simulink library "PC_GS_SSMB"  (R2024a)
settings: Solver=VariableStepAuto  StartTime=0.0  StopTime=10.0  RelTol=1e-3
undefined symbols (not defined in the file): points, X, Y, Z, z_query
libraries: sm_lib x22
settings Model: Creator=jjansev  LastModifiedBy=jjansev

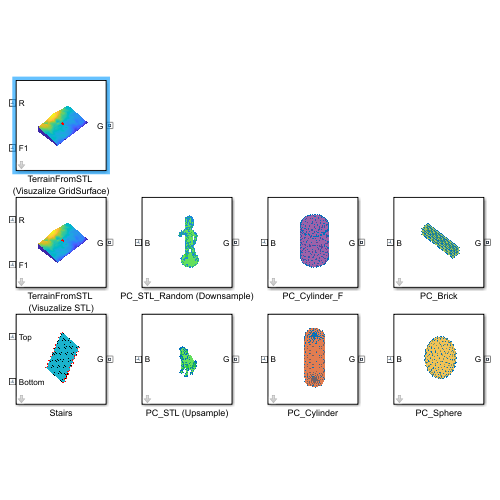
[thumbnail: Simulink's stored preview of the top-level diagram]
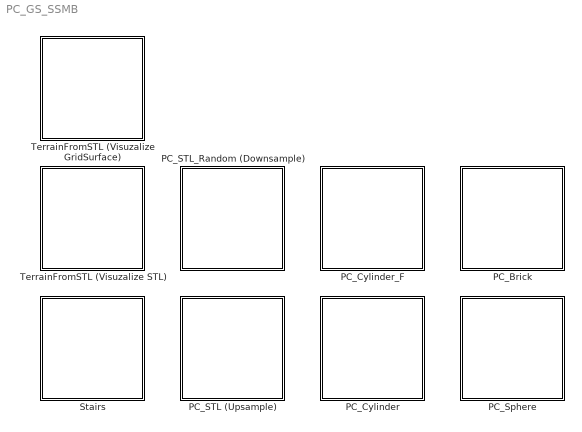
== system PC_GS_SSMB ==
  PC_Brick : Subsystem  mask{length=250, width=50, height=30, numDivisionsLength=25, numDivisionsWidth=5, numDivisionsHeight=3, patchColor=[0.4660, 0.6740, 0.1880], markerColor=[0 0.4470 0.7410]}
      mask prompts: length "Length of the brick (x) [mm]"; width "Width of the brick (y) [mm]"; height "Height of the brick (z) [mm]"; numDivisionsLength "Number of divisions along the length"; numDivisionsWidth "Number of divisions along the width"; numDivisionsHeight "Number of divisions along the height"; patchColor "Color of the patches"; markerColor "Color of the markers"
      mask init:
      | [points, imageMatrix] = generateBrickPointCloud(length, width, height, numDivisionsLength, numDivisionsWidth, numDivisionsHeight, patchColor, markerColor);
      mask Display: image(imageMatrix);
  PC_Cylinder : Subsystem  mask{radius=51, height=200, numRadialDivisions=5, angularOffset=pi/5, numHeightDivisions=25, numFaceRadialDivisions=10, faceAngularOffset=pi/10, numFaceAngularDivisions=10, patchColor=[0.8500, 0.3250, 0.0980], markerColor=[0 0.4470 0.7410]}
      mask prompts: radius "Radius of the cylider [mm]"; height "Height of the cylinder [mm]"; numRadialDivisions "Number of divisions around the circumference"; angularOffset "Angular offset in radians for each layer"; numHeightDivisions "Number of divisions along the height"; numFaceRadialDivisions "Number of radial divisions for the circular faces"; numFaceAngularDivisions "Number of angular divisions for the circular faces"; patchColor "RGB color for the patches"; markerColor "RGB color for the markers"
      mask init:
      | [points, imageMatrix] = generateCylinderPointCloud(radius, height, numRadialDivisions, numHeightDivisions, numFaceRadialDivisions, numFaceAngularDivisions, angularOffset, faceAngularOffset, patchColor, markerColor);
      mask Display: image(imageMatrix);
  PC_Cylinder_F : Subsystem  mask{radius=150/2, height=150, numPoints=150, numCircumferencePoints=50, numFacePoints=50, patchColor=[0.4940, 0.1840, 0.5560], markerColor=[0 0.4470 0.7410]}
      mask prompts: radius "Radius of the cylider [mm]"; height "Height of the cylinder [mm]"; numPoints "Total number of points for the curved surface using the Fibonacci lattice"; numCircumferencePoints "Number of points on the circumference of each disc"; numFacePoints "Number of points on each disc surface using the Fibonacci lattice"; patchColor "RGB color for the patches"; markerColor "RGB color for the markers"
      mask init:
      | [points, imageMatrix] = generateCylinderPointCloudFibonacci(radius, height, numPoints, numCircumferencePoints, numFacePoints, patchColor, markerColor);
      mask Display: image(imageMatrix);
  PC_STL (Upsample) : Subsystem  mask{stlFilename='Low_Poly_Pug.STL', numPoints=0, patchColor=[0.1940, 0.840, 0.1560], markerColor=[0 0.4470 0.7410], STL_points=on}
      mask prompts: stlFilename "Path to the STL file"; numPoints "Number of Points to add inbetween the vertices of the STL"; patchColor "RGB color for the patches"; markerColor "RGB color for the markers"; STL_points "Should the Original STL Points be included in the Point Cloud"
      mask init:
      | % Use set_param to set the parameter
      | fileSolidName = [gcb, '/File Solid'];
      | set_param(fileSolidName, 'ExtGeomFileName', stlFilename);
      | 
      | [points, imageMatrix] = generateSTLPointCloud(stlFilename, numPoints, patchColor, markerColor, STL_points);
      mask Display: image(imageMatrix);
  PC_STL_Random (Downsample) : Subsystem  mask{stlFilename='VaultBoy.STL', numPoints=0, patchColor=[0.1940, 0.840, 0.1560], markerColor=[0.1 0.5470 0.8410], STL_points=on, numPoints2=500}
      mask prompts: stlFilename "Path to the STL file"; numPoints "Points to be added into large surfaces"; patchColor "RGB color for the patches"; markerColor "RGB color for the markers"; STL_points "Should a Subset of the Original STL Points be included in the Point Cloud"; numPoints2 "How many points should be randomly added"
      mask init:
      | % Use set_param to set the parameter
      | fileSolidName = [gcb, '/File Solid'];
      | set_param(fileSolidName, 'ExtGeomFileName', stlFilename);
      | 
      | [points, imageMatrix] = generateSTLPointCloudRandom(stlFilename, numPoints, patchColor, markerColor, STL_points, numPoints2);
      mask Display: image(imageMatrix);
  PC_Sphere : Subsystem  mask{numPoints=256, radius=50, patchColor=[0.9290, 0.6940, 0.1250], markerColor=[0 0.4470 0.7410], dens=1}
      mask prompts: numPoints "Number of points on the Surface of the Sphere"; radius "Radius of the Sphere [mm]"; patchColor "Color of the patches"; markerColor "Color of the markers"; dens "Density"
      mask init:
      | [points, imageMatrix] = generateSpherePointCloud(numPoints, radius, patchColor, markerColor);
      mask Display: image(imageMatrix);
  Stairs : Subsystem  mask{nSteps=10, Tread=180, NosingProtusion=35, Riser=180, yWidth=2000, input_angle_degrees=-45, markerColor=[1 0 0], patchColor=[0.1 0.7 0.8]}
      mask prompts: nSteps "Number of steps"; Tread "Tread [mm]"; NosingProtusion "Nosing Protusion [mm]"; Riser "Riser [mm]"; yWidth "Width of the Staircase"; input_angle_degrees "Degrees to rotate to ensure a single z value per x value [deg]"; markerColor "Color of the markers in the mask image"; patchColor "Surface color"
      mask init:
      | [X_grid_vector, Y_grid_vector, Z_heights, imageMatrix, x, z] = generateStaircaseSurface(nSteps, Tread, NosingProtusion, Riser, yWidth, input_angle_degrees, markerColor, patchColor);
      mask Display: image(imageMatrix);
  TerrainFromSTL (Visuzalize GridSurface) : Subsystem  mask{stlFileName='MRC_t.stl', resolution=1, color=[0.5 0.5 0.6], x_query=0, y_query=0, Int_method=Linear}
      mask prompts: stlFileName "STL Filename"; resolution "Resolution of the Grid surface [m]"; color "Color of the Grid-surface"; x_query "Position on x-axis to be polled for z-height (Frame F1)"; y_query "Position on y-axis to be polled for z-height (Frame F1)"; Int_method "Interpolation method Used of the Surface"
      mask init:
      | % Use set_param to set the parameter
      | fileSolidName = [gcb, '/File Solid'];
      | set_param(fileSolidName, 'ExtGeomFileName', stlFileName);
      | 
      | [imageMatrix, xi, yi, ZI, Res_orig, z_query] = GenerateTerrainFromSTL(stlFileName, resolution, x_query, y_query, Int_method);
      mask Display: image(imageMatrix);
  TerrainFromSTL (Visuzalize STL) : Subsystem  mask{stlFileName='MRC_t.stl', resolution=1, color=[0.5 0.5 0.6], x_query=0, y_query=0, Int_method=Linear}
      mask prompts: stlFileName "STL Filename"; resolution "Resolution of the Grid surface [m]"; color "Color of the Grid-surface"; x_query "Position on x-axis to be polled for z-height (Frame F1)"; y_query "Position on y-axis to be polled for z-height (Frame F1)"; Int_method "Interpolation method Used of the Surface"
      mask init: same as PC_GS_SSMB/TerrainFromSTL (Visuzalize GridSurface)
      mask Display: image(imageMatrix);

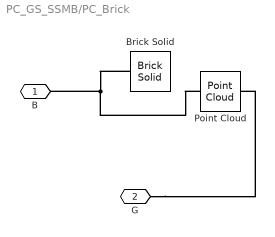
== system PC_GS_SSMB/PC_Brick ==
  Brick Solid : sm_lib/Body Elements/Brick Solid  BrickDimensions=[length width height]  BrickDimensionsUnits=mm  ExportEntireGeometry=off  InertiaType=CalculateFromGeometry  BasedOnType=Density  Density=1000  DensityUnits=kg/m^3  Mass=1  MassUnits=kg  CenterOfMass=[0 0 0]  CenterOfMassUnits=m  MomentsOfInertia=[1 1 1]  MomentsOfInertiaUnits=kg*m^2  ProductsOfInertia=[0 0 0]  ProductsOfInertiaUnits=kg*m^2  GraphicType=FromGeometry  MarkerShape=Sphere  MarkerSize=10  GraphicVisPropType=SimpleVisualProperties  GraphicDiffuseColor=patchColor  GraphicOpacity=0.85  GraphicSpecularColor=[0.5 0.5 0.5 1.0]  GraphicAmbientColor=[0.15 0.15 0.15 1.0]  GraphicEmissiveColor=[0.0 0.0 0.0 1.0]  GraphicShininess=75  DoExposeReferenceFrame=on  SerializedFrames=<Frames/>
  Point Cloud : sm_lib/Curves and Surfaces/Point Cloud  CoordinatesMatrix=points  CoordinatesMatrixUnits=mm  GraphicType=MarkerCloud  GraphicSphereRadius=max(max(points)-min(points))/100*2  GraphicSphereRadiusUnits=mm  GraphicVisPropType=SimpleVisualProperties  GraphicDiffuseColor=markerColor  GraphicOpacity=1  GraphicSpecularColor=[0.5 0.5 0.5 1.0]  GraphicAmbientColor=[0.15 0.15 0.15 1.0]  GraphicEmissiveColor=[0.0 0.0 0.0 1.0]  GraphicShininess=75
  B : PMIOPort  Side=Left
  G : PMIOPort  Port=2  Side=Right
  connections:
  G/RConn1 -- Point Cloud/RConn1
  Point Cloud/LConn1 -- B/RConn1 -- Brick Solid/RConn1

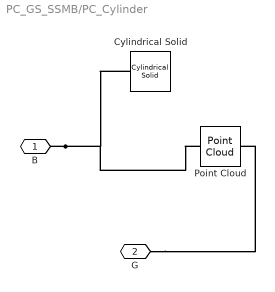
== system PC_GS_SSMB/PC_Cylinder ==
  Cylindrical Solid : sm_lib/Body Elements/Cylindrical Solid  CylinderRadius=radius  CylinderRadiusUnits=mm  CylinderLength=height  CylinderLengthUnits=mm  ExportEntireGeometry=off  InertiaType=CalculateFromGeometry  BasedOnType=Density  Density=1000  DensityUnits=kg/m^3  Mass=1  MassUnits=kg  CenterOfMass=[0 0 0]  CenterOfMassUnits=m  MomentsOfInertia=[1 1 1]  MomentsOfInertiaUnits=kg*m^2  ProductsOfInertia=[0 0 0]  ProductsOfInertiaUnits=kg*m^2  GraphicType=FromGeometry  MarkerShape=Sphere  MarkerSize=10  GraphicVisPropType=SimpleVisualProperties  GraphicDiffuseColor=patchColor  GraphicOpacity=0.85  GraphicSpecularColor=[0.5 0.5 0.5 1.0]  GraphicAmbientColor=[0.15 0.15 0.15 1.0]  GraphicEmissiveColor=[0.0 0.0 0.0 1.0]  GraphicShininess=75  DoExposeReferenceFrame=on  SerializedFrames=<Frames/>
  Point Cloud : sm_lib/Curves and Surfaces/Point Cloud  CoordinatesMatrix=points  CoordinatesMatrixUnits=mm  GraphicType=MarkerCloud  GraphicSphereRadius=max(max(points)-min(points))/100*2  GraphicSphereRadiusUnits=mm  GraphicVisPropType=SimpleVisualProperties  GraphicDiffuseColor=markerColor  GraphicOpacity=1  GraphicSpecularColor=[0.5 0.5 0.5 1.0]  GraphicAmbientColor=[0.15 0.15 0.15 1.0]  GraphicEmissiveColor=[0.0 0.0 0.0 1.0]  GraphicShininess=75
  B : PMIOPort  Side=Left
  G : PMIOPort  Port=2  Side=Right
  connections:
  B/RConn1 -- Point Cloud/LConn1 -- Cylindrical Solid/RConn1
  G/RConn1 -- Point Cloud/RConn1

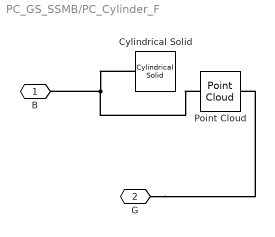
== system PC_GS_SSMB/PC_Cylinder_F ==
  Cylindrical Solid : sm_lib/Body Elements/Cylindrical Solid  CylinderRadius=radius  CylinderRadiusUnits=mm  CylinderLength=height  CylinderLengthUnits=mm  ExportEntireGeometry=off  InertiaType=CalculateFromGeometry  BasedOnType=Density  Density=1000  DensityUnits=kg/m^3  Mass=1  MassUnits=kg  CenterOfMass=[0 0 0]  CenterOfMassUnits=m  MomentsOfInertia=[1 1 1]  MomentsOfInertiaUnits=kg*m^2  ProductsOfInertia=[0 0 0]  ProductsOfInertiaUnits=kg*m^2  GraphicType=FromGeometry  MarkerShape=Sphere  MarkerSize=10  GraphicVisPropType=SimpleVisualProperties  GraphicDiffuseColor=patchColor  GraphicOpacity=0.85  GraphicSpecularColor=[0.5 0.5 0.5 1.0]  GraphicAmbientColor=[0.15 0.15 0.15 1.0]  GraphicEmissiveColor=[0.0 0.0 0.0 1.0]  GraphicShininess=75  DoExposeReferenceFrame=on  SerializedFrames=<Frames/>
  Point Cloud : sm_lib/Curves and Surfaces/Point Cloud  CoordinatesMatrix=points  CoordinatesMatrixUnits=mm  GraphicType=MarkerCloud  GraphicSphereRadius=max(max(points)-min(points))/100*2  GraphicSphereRadiusUnits=mm  GraphicVisPropType=SimpleVisualProperties  GraphicDiffuseColor=markerColor  GraphicOpacity=1  GraphicSpecularColor=[0.5 0.5 0.5 1.0]  GraphicAmbientColor=[0.15 0.15 0.15 1.0]  GraphicEmissiveColor=[0.0 0.0 0.0 1.0]  GraphicShininess=75
  B : PMIOPort  Side=Left
  G : PMIOPort  Port=2  Side=Right
  connections:
  G/RConn1 -- Point Cloud/RConn1
  Point Cloud/LConn1 -- B/RConn1 -- Cylindrical Solid/RConn1

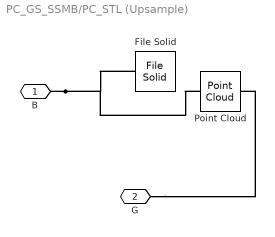
== system PC_GS_SSMB/PC_STL (Upsample) ==
  File Solid : sm_lib/Body Elements/File Solid  ExtGeomFileName=Low_Poly_Pug.STL  UnitType=Custom  ExtGeomFileUnits=mm  StepReaderType=HEX  ExportConvexHullGeometry=off  InertiaType=CalculateFromGeometry  BasedOnType=Density  Density=7850  DensityUnits=kg/m^3  Mass=1  MassUnits=kg  CenterOfMass=[0 0 0]  CenterOfMassUnits=m  MomentsOfInertia=[1 1 1]  MomentsOfInertiaUnits=kg*m^2  ProductsOfInertia=[0 0 0]  ProductsOfInertiaUnits=kg*m^2  GraphicType=FromGeometry  MarkerShape=Sphere  MarkerSize=10  GraphicVisPropType=SimpleVisualProperties  GraphicDiffuseColor=patchColor  GraphicOpacity=1  GraphicSpecularColor=[0.5 0.5 0.5 1.0]  GraphicAmbientColor=[0.15 0.15 0.15 1.0]  GraphicEmissiveColor=[0.0 0.0 0.0 1.0]  GraphicShininess=75  DoExposeReferenceFrame=on  SerializedFrames=<Frames/>
  Point Cloud : sm_lib/Curves and Surfaces/Point Cloud  CoordinatesMatrix=points  CoordinatesMatrixUnits=mm  GraphicType=MarkerCloud  GraphicSphereRadius=max(max(points)-min(points))/100*2  GraphicSphereRadiusUnits=mm  GraphicVisPropType=SimpleVisualProperties  GraphicDiffuseColor=markerColor  GraphicOpacity=1  GraphicSpecularColor=[0.5 0.5 0.5 1.0]  GraphicAmbientColor=[0.15 0.15 0.15 1.0]  GraphicEmissiveColor=[0.0 0.0 0.0 1.0]  GraphicShininess=75
  B : PMIOPort  Side=Left
  G : PMIOPort  Port=2  Side=Right
  connections:
  B/RConn1 -- Point Cloud/LConn1 -- File Solid/RConn1
  G/RConn1 -- Point Cloud/RConn1

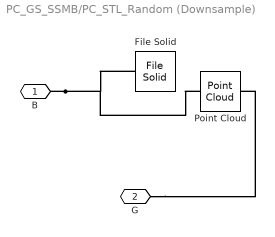
== system PC_GS_SSMB/PC_STL_Random (Downsample) ==
  File Solid : sm_lib/Body Elements/File Solid  ExtGeomFileName=VaultBoy.STL  UnitType=Custom  ExtGeomFileUnits=mm  StepReaderType=HEX  ExportConvexHullGeometry=off  InertiaType=CalculateFromGeometry  BasedOnType=Density  Density=7850  DensityUnits=kg/m^3  Mass=1  MassUnits=kg  CenterOfMass=[0 0 0]  CenterOfMassUnits=m  MomentsOfInertia=[1 1 1]  MomentsOfInertiaUnits=kg*m^2  ProductsOfInertia=[0 0 0]  ProductsOfInertiaUnits=kg*m^2  GraphicType=FromGeometry  MarkerShape=Sphere  MarkerSize=10  GraphicVisPropType=SimpleVisualProperties  GraphicDiffuseColor=patchColor  GraphicOpacity=1  GraphicSpecularColor=[0.5 0.5 0.5 1.0]  GraphicAmbientColor=[0.15 0.15 0.15 1.0]  GraphicEmissiveColor=[0.0 0.0 0.0 1.0]  GraphicShininess=75  DoExposeReferenceFrame=on  SerializedFrames=<Frames/>
  Point Cloud : sm_lib/Curves and Surfaces/Point Cloud  CoordinatesMatrix=points  CoordinatesMatrixUnits=mm  GraphicType=MarkerCloud  GraphicSphereRadius=max(max(points)-min(points))/100*2  GraphicSphereRadiusUnits=mm  GraphicVisPropType=SimpleVisualProperties  GraphicDiffuseColor=markerColor  GraphicOpacity=1  GraphicSpecularColor=[0.5 0.5 0.5 1.0]  GraphicAmbientColor=[0.15 0.15 0.15 1.0]  GraphicEmissiveColor=[0.0 0.0 0.0 1.0]  GraphicShininess=75
  B : PMIOPort  Side=Left
  G : PMIOPort  Port=2  Side=Right
  connections:
  B/RConn1 -- Point Cloud/LConn1 -- File Solid/RConn1
  G/RConn1 -- Point Cloud/RConn1

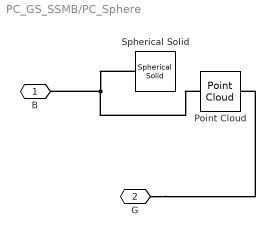
== system PC_GS_SSMB/PC_Sphere ==
  Point Cloud : sm_lib/Curves and Surfaces/Point Cloud  CoordinatesMatrix=points  CoordinatesMatrixUnits=mm  GraphicType=MarkerCloud  GraphicSphereRadius=max(max(points)-min(points))/100*2  GraphicSphereRadiusUnits=mm  GraphicVisPropType=SimpleVisualProperties  GraphicDiffuseColor=markerColor  GraphicOpacity=1  GraphicSpecularColor=[0.5 0.5 0.5 1.0]  GraphicAmbientColor=[0.15 0.15 0.15 1.0]  GraphicEmissiveColor=[0.0 0.0 0.0 1.0]  GraphicShininess=75
  Spherical Solid : sm_lib/Body Elements/Spherical Solid  SphereRadius=radius  SphereRadiusUnits=mm  ExportEntireGeometry=off  InertiaType=CalculateFromGeometry  BasedOnType=Density  Density=dens  DensityUnits=kg/m^3  Mass=1  MassUnits=kg  CenterOfMass=[0 0 0]  CenterOfMassUnits=m  MomentsOfInertia=[1 1 1]  MomentsOfInertiaUnits=kg*m^2  ProductsOfInertia=[0 0 0]  ProductsOfInertiaUnits=kg*m^2  GraphicType=FromGeometry  MarkerShape=Sphere  MarkerSize=10  GraphicVisPropType=SimpleVisualProperties  GraphicDiffuseColor=patchColor  GraphicOpacity=0.85  GraphicSpecularColor=[0.5 0.5 0.5 1.0]  GraphicAmbientColor=[0.15 0.15 0.15 1.0]  GraphicEmissiveColor=[0.0 0.0 0.0 1.0]  GraphicShininess=75  DoExposeReferenceFrame=on  SerializedFrames=<Frames/>
  B : PMIOPort  Side=Left
  G : PMIOPort  Port=2  Side=Right
  connections:
  Spherical Solid/RConn1 -- B/RConn1 -- Point Cloud/LConn1
  G/RConn1 -- Point Cloud/RConn1

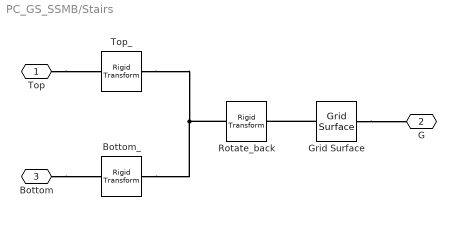
== system PC_GS_SSMB/Stairs ==
  Bottom_ : sm_lib/Frames and Transforms/Rigid Transform  RotationMethod=None  FollAlignAxisA=+X  BaseAlignAxisA=+Y  FollAlignAxisB=+Y  BaseAlignAxisB=+Z  RotationStandardAxis=-Y  RotationAngle=45  RotationAngleUnits=deg  RotationArbitraryAxis=[0 0 1]  RotationSequenceAxes=FollowerAxes  RotationSequence=XYX  RotationSequenceAngles=[0 0 0]  RotationSequenceAnglesUnits=deg  RotationMatrix=[1 0 0; 0 1 0; 0 0 1]  Quaternion=[1 0 0 0]  TranslationMethod=Cartesian  TranslationCartesianOffset=[0 -yWidth/2 0]  TranslationCartesianOffsetUnits=mm  TranslationStandardAxis=+Z  TranslationStandardOffset=0  TranslationStandardOffsetUnits=m  TranslationROffset=0  TranslationROffsetUnits=m  TranslationThetaOffset=0  TranslationThetaOffsetUnits=deg  TranslationZOffset=0  TranslationZOffsetUnits=m
  Grid Surface : sm_lib/Curves and Surfaces/Grid Surface  XGridVector=X_grid_vector  XGridVectorUnits=mm  YGridVector=Y_grid_vector  YGridVectorUnits=mm  ZHeights=Z_heights'  ZHeightsUnits=mm  GraphicType=FromGeometry  GraphicVisPropType=SimpleVisualProperties  GraphicDiffuseColor=patchColor  GraphicOpacity=1  GraphicSpecularColor=[0.5 0.5 0.5 1.0]  GraphicAmbientColor=[0.15 0.15 0.15 1.0]  GraphicEmissiveColor=[0.0 0.0 0.0 1.0]  GraphicShininess=75
  Rotate_back : sm_lib/Frames and Transforms/Rigid Transform  RotationMethod=StandardAxis  FollAlignAxisA=+X  BaseAlignAxisA=+Y  FollAlignAxisB=+Y  BaseAlignAxisB=+Z  RotationStandardAxis=-Y  RotationAngle=45  RotationAngleUnits=deg  RotationArbitraryAxis=[0 0 1]  RotationSequenceAxes=FollowerAxes  RotationSequence=XYX  RotationSequenceAngles=[0 0 0]  RotationSequenceAnglesUnits=deg  RotationMatrix=[1 0 0; 0 1 0; 0 0 1]  Quaternion=[1 0 0 0]  TranslationMethod=Cartesian  TranslationCartesianOffset=[0 -yWidth/2 0]  TranslationCartesianOffsetUnits=mm  TranslationStandardAxis=+Z  TranslationStandardOffset=0  TranslationStandardOffsetUnits=m  TranslationROffset=0  TranslationROffsetUnits=m  TranslationThetaOffset=0  TranslationThetaOffsetUnits=deg  TranslationZOffset=0  TranslationZOffsetUnits=m
  Top_ : sm_lib/Frames and Transforms/Rigid Transform  RotationMethod=None  FollAlignAxisA=+X  BaseAlignAxisA=+Y  FollAlignAxisB=+Y  BaseAlignAxisB=+Z  RotationStandardAxis=-Y  RotationAngle=45  RotationAngleUnits=deg  RotationArbitraryAxis=[0 0 1]  RotationSequenceAxes=FollowerAxes  RotationSequence=XYX  RotationSequenceAngles=[0 0 0]  RotationSequenceAnglesUnits=deg  RotationMatrix=[1 0 0; 0 1 0; 0 0 1]  Quaternion=[1 0 0 0]  TranslationMethod=Cartesian  TranslationCartesianOffset=[x(end) 0 z(end)]  TranslationCartesianOffsetUnits=mm  TranslationStandardAxis=+Z  TranslationStandardOffset=0  TranslationStandardOffsetUnits=m  TranslationROffset=0  TranslationROffsetUnits=m  TranslationThetaOffset=0  TranslationThetaOffsetUnits=deg  TranslationZOffset=0  TranslationZOffsetUnits=m
  Top : PMIOPort  Side=Left
  G : PMIOPort  Port=2  Side=Right
  Bottom : PMIOPort  Port=3  Side=Left
  connections:
  Grid Surface/LConn1 -- Rotate_back/RConn1
  Rotate_back/LConn1 -- Bottom_/LConn1 -- Top_/LConn1
  Grid Surface/RConn1 -- G/RConn1
  Top/RConn1 -- Top_/RConn1
  Bottom/RConn1 -- Bottom_/RConn1

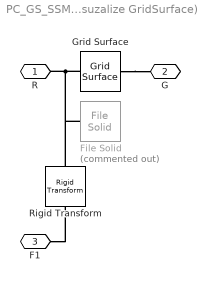
== system PC_GS_SSMB/TerrainFromSTL (Visuzalize GridSurface) ==
  File Solid : sm_lib/Body Elements/File Solid  Commented=on  ExtGeomFileName=MRC_t.stl  UnitType=Custom  ExtGeomFileUnits=m  StepReaderType=HEX  ExportConvexHullGeometry=off  InertiaType=PointMass  BasedOnType=DensityFromFile  Density=1000  DensityUnits=kg/m^3  Mass=0  MassUnits=kg  CenterOfMass=[0 0 0]  CenterOfMassUnits=m  MomentsOfInertia=[1 1 1]  MomentsOfInertiaUnits=kg*m^2  ProductsOfInertia=[0 0 0]  ProductsOfInertiaUnits=kg*m^2  GraphicType=FromGeometry  MarkerShape=Sphere  MarkerSize=10  GraphicVisPropType=SimpleVisualProperties  GraphicDiffuseColor=color  GraphicOpacity=1  GraphicSpecularColor=[0.5 0.5 0.5 1.0]  GraphicAmbientColor=[0.15 0.15 0.15 1.0]  GraphicEmissiveColor=[0.0 0.0 0.0 1.0]  GraphicShininess=75  DoExposeReferenceFrame=on  SerializedFrames=<Frames/>
  Grid Surface : sm_lib/Curves and Surfaces/Grid Surface  XGridVector=xi'  XGridVectorUnits=m  YGridVector=yi'  YGridVectorUnits=m  ZHeights=ZI'  ZHeightsUnits=m  GraphicType=FromGeometry  GraphicVisPropType=SimpleVisualProperties  GraphicDiffuseColor=color  GraphicOpacity=1  GraphicSpecularColor=[0.5 0.5 0.5 1.0]  GraphicAmbientColor=[0.15 0.15 0.15 1.0]  GraphicEmissiveColor=[0.0 0.0 0.0 1.0]  GraphicShininess=75
  Rigid Transform : sm_lib/Frames and Transforms/Rigid Transform  RotationMethod=None  FollAlignAxisA=+X  BaseAlignAxisA=+Y  FollAlignAxisB=+Y  BaseAlignAxisB=+Z  RotationStandardAxis=+Z  RotationAngle=0  RotationAngleUnits=deg  RotationArbitraryAxis=[0 0 1]  RotationSequenceAxes=FollowerAxes  RotationSequence=XYX  RotationSequenceAngles=[0 0 0]  RotationSequenceAnglesUnits=deg  RotationMatrix=[1 0 0;0 1 0;0 0 1]  Quaternion=[1 0 0 0]  TranslationMethod=Cartesian  TranslationCartesianOffset=[x_query y_query z_query]  TranslationCartesianOffsetUnits=m  TranslationStandardAxis=+Z  TranslationStandardOffset=0  TranslationStandardOffsetUnits=m  TranslationROffset=0  TranslationROffsetUnits=m  TranslationThetaOffset=0  TranslationThetaOffsetUnits=deg  TranslationZOffset=0  TranslationZOffsetUnits=m
  R : PMIOPort  Side=Left
  G : PMIOPort  Port=2  Side=Right
  F1 : PMIOPort  Port=3  Side=Left
  connections:
  F1/RConn1 -- Rigid Transform/RConn1
  Grid Surface/LConn1 -- File Solid/RConn1 -- Rigid Transform/LConn1 -- R/RConn1
  Grid Surface/RConn1 -- G/RConn1

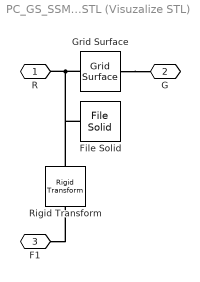
== system PC_GS_SSMB/TerrainFromSTL (Visuzalize STL) ==
  File Solid : sm_lib/Body Elements/File Solid  ExtGeomFileName=MRC_t.stl  UnitType=Custom  ExtGeomFileUnits=m  StepReaderType=HEX  ExportConvexHullGeometry=off  InertiaType=PointMass  BasedOnType=DensityFromFile  Density=1000  DensityUnits=kg/m^3  Mass=0  MassUnits=kg  CenterOfMass=[0 0 0]  CenterOfMassUnits=m  MomentsOfInertia=[1 1 1]  MomentsOfInertiaUnits=kg*m^2  ProductsOfInertia=[0 0 0]  ProductsOfInertiaUnits=kg*m^2  GraphicType=FromGeometry  MarkerShape=Sphere  MarkerSize=10  GraphicVisPropType=SimpleVisualProperties  GraphicDiffuseColor=color  GraphicOpacity=1  GraphicSpecularColor=[0.5 0.5 0.5 1.0]  GraphicAmbientColor=[0.15 0.15 0.15 1.0]  GraphicEmissiveColor=[0.0 0.0 0.0 1.0]  GraphicShininess=75  DoExposeReferenceFrame=on  SerializedFrames=<Frames/>
  Grid Surface : sm_lib/Curves and Surfaces/Grid Surface  XGridVector=xi'  XGridVectorUnits=m  YGridVector=yi'  YGridVectorUnits=m  ZHeights=ZI'  ZHeightsUnits=m  GraphicType=None  GraphicVisPropType=SimpleVisualProperties  GraphicDiffuseColor=color  GraphicOpacity=1  GraphicSpecularColor=[0.5 0.5 0.5 1.0]  GraphicAmbientColor=[0.15 0.15 0.15 1.0]  GraphicEmissiveColor=[0.0 0.0 0.0 1.0]  GraphicShininess=75
  Rigid Transform : sm_lib/Frames and Transforms/Rigid Transform  RotationMethod=None  FollAlignAxisA=+X  BaseAlignAxisA=+Y  FollAlignAxisB=+Y  BaseAlignAxisB=+Z  RotationStandardAxis=+Z  RotationAngle=0  RotationAngleUnits=deg  RotationArbitraryAxis=[0 0 1]  RotationSequenceAxes=FollowerAxes  RotationSequence=XYX  RotationSequenceAngles=[0 0 0]  RotationSequenceAnglesUnits=deg  RotationMatrix=[1 0 0;0 1 0;0 0 1]  Quaternion=[1 0 0 0]  TranslationMethod=Cartesian  TranslationCartesianOffset=[x_query y_query z_query]  TranslationCartesianOffsetUnits=m  TranslationStandardAxis=+Z  TranslationStandardOffset=0  TranslationStandardOffsetUnits=m  TranslationROffset=0  TranslationROffsetUnits=m  TranslationThetaOffset=0  TranslationThetaOffsetUnits=deg  TranslationZOffset=0  TranslationZOffsetUnits=m
  R : PMIOPort  Side=Left
  G : PMIOPort  Port=2  Side=Right
  F1 : PMIOPort  Port=3  Side=Left
  connections:
  F1/RConn1 -- Rigid Transform/RConn1
  Grid Surface/LConn1 -- File Solid/RConn1 -- Rigid Transform/LConn1 -- R/RConn1
  Grid Surface/RConn1 -- G/RConn1
